simulink model "tres_test_multikernel"  (R2014a)
settings: Solver=VariableStepDiscrete  StartTime=0.0  StopTime=120  RelTol=1e-3
libraries: tres_simulink_blockset x9
settings Model: Creator=matteo  LastModifiedBy=MM244911
settings DataIOCC: SignalLoggingSaveFormat=ModelDataLogs
settings OptimizationCC: ExpressionDepthLimit=2147483647
settings DebuggingCC: UnderspecifiedInitializationDetection=Classic  FcnCallInpInsideContextMsg=EnableAllAsWarning  StateNameClashWarn=warning

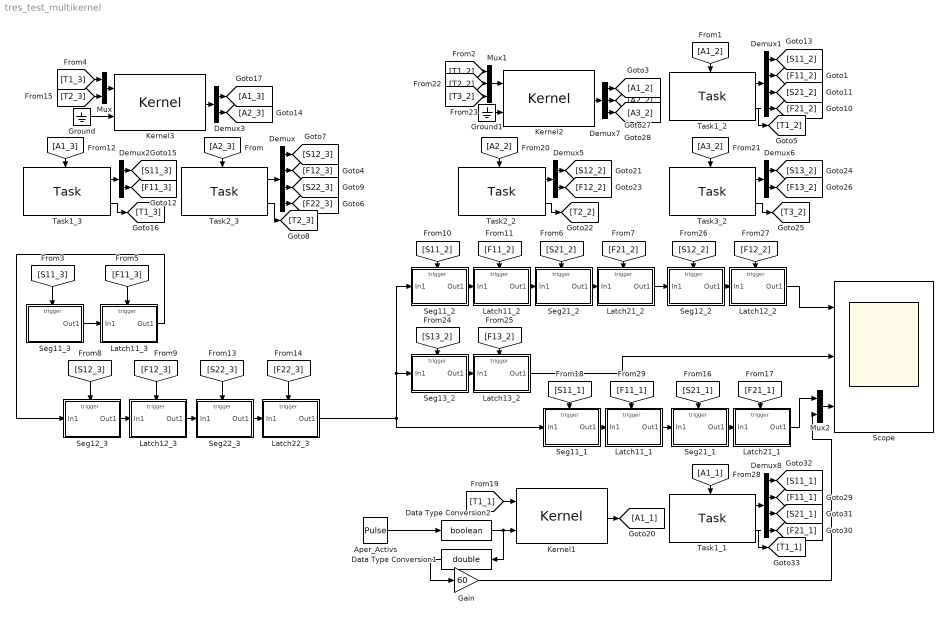
== system tres_test_multikernel ==
  Aper_Activs : DiscretePulseGenerator  PulseType=Time based  Period=15  PulseWidth=100/15  PhaseDelay=15
  Data Type Conversion1 : DataTypeConversion  OutDataTypeStr=double
  Data Type Conversion2 : DataTypeConversion  OutDataTypeStr=boolean
  Demux : Demux
  Demux1 : Demux
  Demux{2..3,5..6} (4 alike) : Demux  Outputs=2
  Demux7 : Demux  Outputs=3
  Demux8 : Demux
  Gain : Gain  Gain=60
  Ground : Ground
  Ground1 : Ground
  Kernel1 : tres_simulink_blockset/Kernel  taskset_descr_name=task_set_descr1  scheduling_policy=DEADLINE_MONOTONIC  dead_miss_rule=Continue  time_res=Milli_Seconds  core_num=1  under_engine=RTSIM
  Kernel2 : tres_simulink_blockset/Kernel  taskset_descr_name=task_set_descr2  scheduling_policy=DEADLINE_MONOTONIC  dead_miss_rule=Continue  time_res=Milli_Seconds  core_num=2  under_engine=RTSIM
  Kernel3 : tres_simulink_blockset/Kernel  taskset_descr_name=task_set_descr3  scheduling_policy=DEADLINE_MONOTONIC  dead_miss_rule=Continue  time_res=Milli_Seconds  core_num=1  under_engine=RTSIM
  Latch11_1 : Subsystem  TreatAsAtomicUnit=on
  Latch11_2 : Subsystem  TreatAsAtomicUnit=on
  Latch11_3 : Subsystem  TreatAsAtomicUnit=on
  Latch12_2 : Subsystem  TreatAsAtomicUnit=on
  Latch12_3 : Subsystem  TreatAsAtomicUnit=on
  Latch13_2 : Subsystem  TreatAsAtomicUnit=on
  Latch21_1 : Subsystem  TreatAsAtomicUnit=on
  Latch21_2 : Subsystem  TreatAsAtomicUnit=on
  Latch22_3 : Subsystem  TreatAsAtomicUnit=on
  Mux : Mux  Inputs=2
  Mux1 : Mux  Inputs=3
  Mux2 : Mux  Inputs=2
  Scope : Scope  NumInputPorts=3
      settings: YMin=-5~-5~-5  YMax=5~5~5
  Seg11_1 : Subsystem  TreatAsAtomicUnit=on
  Seg11_2 : Subsystem  TreatAsAtomicUnit=on
  Seg11_3 : Subsystem  TreatAsAtomicUnit=on
  Seg12_2 : Subsystem  TreatAsAtomicUnit=on
  Seg12_3 : Subsystem  TreatAsAtomicUnit=on
  Seg13_2 : Subsystem  TreatAsAtomicUnit=on
  Seg21_1 : Subsystem  TreatAsAtomicUnit=on
  Seg21_2 : Subsystem  TreatAsAtomicUnit=on
  Seg22_3 : Subsystem  TreatAsAtomicUnit=on
  Task1_1 : tres_simulink_blockset/Task  conf_name=t11_instrs
  Task1_2 : tres_simulink_blockset/Task  conf_name=t12_instrs
  Task1_3 : tres_simulink_blockset/Task  conf_name=t13_instrs
  Task2_2 : tres_simulink_blockset/Task  conf_name=t22_instrs
  Task2_3 : tres_simulink_blockset/Task  conf_name=t23_instrs
  Task3_2 : tres_simulink_blockset/Task  conf_name=t32_instrs
  wires:
  Task1_2/2 -> [T1_2]
  Task2_3/2 -> [T2_3]
  Seg11_3/1(Out1) -> Latch11_3/1(In1)
  Seg21_2/1(Out1) -> Latch21_2/1(In1)
  Ground/1 -> Kernel3/2
  Demux/1 -> [S12_3]
  Demux/2 -> [F12_3]
  Task2_3/1 -> Demux/1
  Task1_2/1 -> Demux1/1
  [A2_3] -> Task2_3/Trigger
  [A1_2] -> Task1_2/Trigger
  Kernel3/1 -> Demux3/1
  Ground1/1 -> Kernel2/2
  [S11_3] -> Seg11_3/Trigger
  [F11_3] -> Latch11_3/Trigger
  [S21_2] -> Seg21_2/Trigger
  [F21_2] -> Latch21_2/Trigger
  Demux/4 -> [F22_3]
  Demux/3 -> [S22_3]
  Demux1/1 -> [S11_2]
  Demux1/2 -> [F11_2]
  Demux1/4 -> [F21_2]
  Demux1/3 -> [S21_2]
  Seg12_3/1(Out1) -> Latch12_3/1(In1)
  [F12_3] -> Latch12_3/Trigger
  [S12_3] -> Seg12_3/Trigger
  Latch11_3/1(Out1) -> Seg12_3/1(In1)
  Seg11_2/1(Out1) -> Latch11_2/1(In1)
  [S11_2] -> Seg11_2/Trigger
  [F11_2] -> Latch11_2/Trigger
  Latch11_2/1(Out1) -> Seg21_2/1(In1)
  Task1_3/2 -> [T1_3]
  Demux2/1 -> [S11_3]
  Demux2/2 -> [F11_3]
  Task1_3/1 -> Demux2/1
  [A1_3] -> Task1_3/Trigger
  [F22_3] -> Latch22_3/Trigger
  [S22_3] -> Seg22_3/Trigger
  Latch12_3/1(Out1) -> Seg22_3/1(In1)
  Seg22_3/1(Out1) -> Latch22_3/1(In1)
  Latch22_3/1(Out1) -> Seg11_1/1(In1), Seg13_2/1(In1), Seg11_2/1(In1)
  Demux3/1 -> [A1_3]
  Demux3/2 -> [A2_3]
  [T2_3] -> Mux/2
  [T1_3] -> Mux/1
  Mux/1 -> Kernel3/1
  Seg21_1/1(Out1) -> Latch21_1/1(In1)
  [S21_1] -> Seg21_1/Trigger
  [T1_1] -> Kernel1/1
  Data Type Conversion2/1 -> Data Type Conversion1/1, Kernel1/2
  Kernel1/1 -> [A1_1]
  [F21_1] -> Latch21_1/Trigger
  Task2_2/2 -> [T2_2]
  Demux5/1 -> [S12_2]
  Demux5/2 -> [F12_2]
  Task2_2/1 -> Demux5/1
  [A2_2] -> Task2_2/Trigger
  Task3_2/2 -> [T3_2]
  Demux6/1 -> [S13_2]
  Demux6/2 -> [F13_2]
  Task3_2/1 -> Demux6/1
  [A3_2] -> Task3_2/Trigger
  Mux1/1 -> Kernel2/1
  [T1_2] -> Mux1/1
  [T2_2] -> Mux1/2
  [T3_2] -> Mux1/3
  Seg13_2/1(Out1) -> Latch13_2/1(In1)
  [S13_2] -> Seg13_2/Trigger
  [F13_2] -> Latch13_2/Trigger
  Seg12_2/1(Out1) -> Latch12_2/1(In1)
  [S12_2] -> Seg12_2/Trigger
  [F12_2] -> Latch12_2/Trigger
  Latch13_2/1(Out1) -> Scope/2
  Latch12_2/1(Out1) -> Scope/1
  Latch21_2/1(Out1) -> Seg12_2/1(In1)
  Kernel2/1 -> Demux7/1
  Demux7/1 -> [A1_2]
  Demux7/3 -> [A3_2]
  Demux7/2 -> [A2_2]
  Task1_1/2 -> [T1_1]
  Task1_1/1 -> Demux8/1
  [A1_1] -> Task1_1/Trigger
  Demux8/1 -> [S11_1]
  Demux8/2 -> [F11_1]
  Demux8/4 -> [F21_1]
  Demux8/3 -> [S21_1]
  Seg11_1/1(Out1) -> Latch11_1/1(In1)
  [S11_1] -> Seg11_1/Trigger
  [F11_1] -> Latch11_1/Trigger
  Latch11_1/1(Out1) -> Seg21_1/1(In1)
  Aper_Activs/1 -> Data Type Conversion2/1
  Latch21_1/1(Out1) -> Mux2/1
  Data Type Conversion1/1 -> Gain/1
  Mux2/1 -> Scope/3
  Gain/1 -> Mux2/2

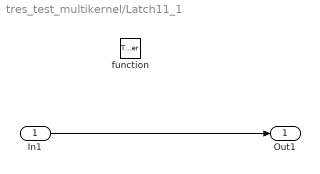
== system tres_test_multikernel/Latch11_1 ==
  In1 : Inport
  function : TriggerPort  TriggerType=function-call
  Out1 : Outport
  wires:
  In1/1 -> Out1/1

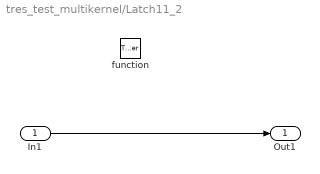
== system tres_test_multikernel/Latch11_2 ==
  In1 : Inport
  function : TriggerPort  TriggerType=function-call
  Out1 : Outport
  wires:
  In1/1 -> Out1/1

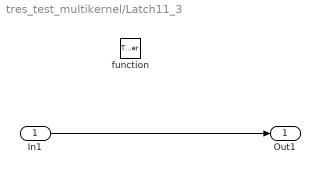
== system tres_test_multikernel/Latch11_3 ==
  In1 : Inport
  function : TriggerPort  TriggerType=function-call
  Out1 : Outport
  wires:
  In1/1 -> Out1/1

== system tres_test_multikernel/Latch12_2 ==
  In1 : Inport
  function : TriggerPort  TriggerType=function-call
  Out1 : Outport
  wires:
  In1/1 -> Out1/1

== system tres_test_multikernel/Latch12_3 ==
  In1 : Inport
  function : TriggerPort  TriggerType=function-call
  Out1 : Outport
  wires:
  In1/1 -> Out1/1

== system tres_test_multikernel/Latch13_2 ==
  In1 : Inport
  function : TriggerPort  TriggerType=function-call
  Out1 : Outport
  wires:
  In1/1 -> Out1/1

== system tres_test_multikernel/Latch21_1 ==
  In1 : Inport
  function : TriggerPort  TriggerType=function-call
  Out1 : Outport
  wires:
  In1/1 -> Out1/1

== system tres_test_multikernel/Latch21_2 ==
  In1 : Inport
  function : TriggerPort  TriggerType=function-call
  Out1 : Outport
  wires:
  In1/1 -> Out1/1

== system tres_test_multikernel/Latch22_3 ==
  In1 : Inport
  function : TriggerPort  TriggerType=function-call
  Out1 : Outport
  wires:
  In1/1 -> Out1/1

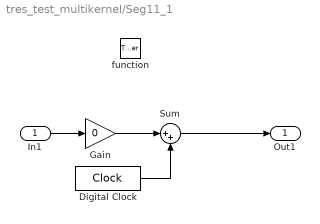
== system tres_test_multikernel/Seg11_1 ==
  In1 : Inport
  function : TriggerPort  TriggerType=function-call
  Digital Clock : DigitalClock  SampleTime=-1
  Gain : Gain  Gain=0
  Sum : Sum  Inputs=|++
  Out1 : Outport
  wires:
  Sum/1 -> Out1/1
  Digital Clock/1 -> Sum/2
  In1/1 -> Gain/1
  Gain/1 -> Sum/1

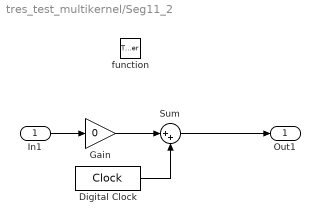
== system tres_test_multikernel/Seg11_2 ==
  In1 : Inport
  function : TriggerPort  TriggerType=function-call
  Digital Clock : DigitalClock  SampleTime=-1
  Gain : Gain  Gain=0
  Sum : Sum  Inputs=|++
  Out1 : Outport
  wires:
  Sum/1 -> Out1/1
  Digital Clock/1 -> Sum/2
  In1/1 -> Gain/1
  Gain/1 -> Sum/1

== system tres_test_multikernel/Seg11_3 ==
  function : TriggerPort  TriggerType=function-call
  Digital Clock : DigitalClock  SampleTime=-1
  Out1 : Outport
  wires:
  Digital Clock/1 -> Out1/1

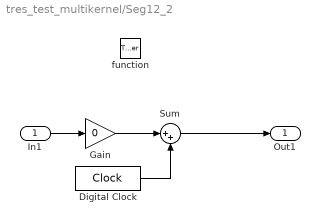
== system tres_test_multikernel/Seg12_2 ==
  In1 : Inport
  function : TriggerPort  TriggerType=function-call
  Digital Clock : DigitalClock  SampleTime=-1
  Gain : Gain  Gain=0
  Sum : Sum  Inputs=|++
  Out1 : Outport
  wires:
  Sum/1 -> Out1/1
  Digital Clock/1 -> Sum/2
  In1/1 -> Gain/1
  Gain/1 -> Sum/1

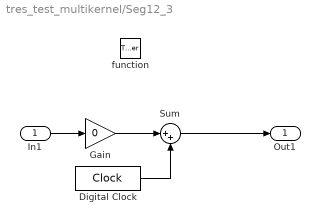
== system tres_test_multikernel/Seg12_3 ==
  In1 : Inport
  function : TriggerPort  TriggerType=function-call
  Digital Clock : DigitalClock  SampleTime=-1
  Gain : Gain  Gain=0
  Sum : Sum  Inputs=|++
  Out1 : Outport
  wires:
  Sum/1 -> Out1/1
  Digital Clock/1 -> Sum/2
  In1/1 -> Gain/1
  Gain/1 -> Sum/1

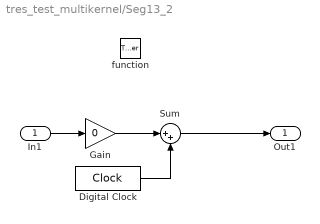
== system tres_test_multikernel/Seg13_2 ==
  In1 : Inport
  function : TriggerPort  TriggerType=function-call
  Digital Clock : DigitalClock  SampleTime=-1
  Gain : Gain  Gain=0
  Sum : Sum  Inputs=|++
  Out1 : Outport
  wires:
  Sum/1 -> Out1/1
  Digital Clock/1 -> Sum/2
  In1/1 -> Gain/1
  Gain/1 -> Sum/1

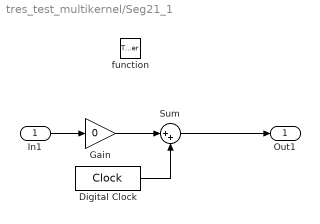
== system tres_test_multikernel/Seg21_1 ==
  In1 : Inport
  function : TriggerPort  TriggerType=function-call
  Digital Clock : DigitalClock  SampleTime=-1
  Gain : Gain  Gain=0
  Sum : Sum  Inputs=|++
  Out1 : Outport
  wires:
  Sum/1 -> Out1/1
  Digital Clock/1 -> Sum/2
  In1/1 -> Gain/1
  Gain/1 -> Sum/1

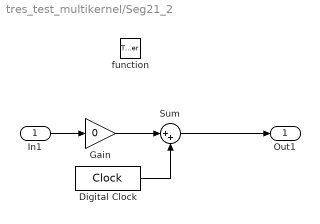
== system tres_test_multikernel/Seg21_2 ==
  In1 : Inport
  function : TriggerPort  TriggerType=function-call
  Digital Clock : DigitalClock  SampleTime=-1
  Gain : Gain  Gain=0
  Sum : Sum  Inputs=|++
  Out1 : Outport
  wires:
  Sum/1 -> Out1/1
  Digital Clock/1 -> Sum/2
  In1/1 -> Gain/1
  Gain/1 -> Sum/1

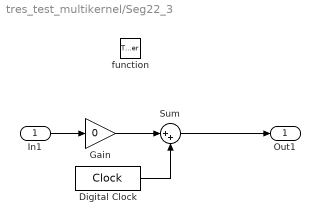
== system tres_test_multikernel/Seg22_3 ==
  In1 : Inport
  function : TriggerPort  TriggerType=function-call
  Digital Clock : DigitalClock  SampleTime=-1
  Gain : Gain  Gain=0
  Sum : Sum  Inputs=|++
  Out1 : Outport
  wires:
  Sum/1 -> Out1/1
  Digital Clock/1 -> Sum/2
  In1/1 -> Gain/1
  Gain/1 -> Sum/1
